simulink model "Iface"  (R2018b)
settings: Solver=FixedStepDiscrete  StartTime=0.0  StopTime=10.0  RelTol=1e-3
settings Model: Creator=matlab  LastModifiedBy=matlab
settings DataIOCC: SaveOutput=off  SignalLogging=off  SaveTime=off
settings OptimizationCC: DefaultParameterBehavior=Inlined  EnhancedBackFolding=on  PassReuseOutputArgsAs=Individual arguments  OptimizeBlockOrder=speed  DifferentSizesBufferReuse=on  OptimizationCustomize=off
settings DebuggingCC: ParameterTunabilityLossMsg=error
settings SFSimCC: MATLABDynamicMemAlloc=off
settings RTWCC: SystemTargetFile=ert.tlc  TemplateMakefile=ert_default_tmf  PostCodeGenCommand=packNGo(buildInfo);  GenerateReport=on  IncludeHyperlinkInReport=on  LaunchReport=on  GenerateTraceInfo=on  GenerateTraceReport=on  GenerateTraceReportSl=on  GenerateTraceReportSf=on  GenerateTraceReportEml=on
settings CodeAppCC: ForceParamTrailComments=on  IgnoreCustomStorageClasses=off  OperatorAnnotations=on  SimulinkDataObjDesc=on  SFDataObjDesc=on  InsertBlockDesc=on
settings ERTTargetCC: TargetLangStandard=C99 (ISO)  GenerateSampleERTMain=on  InlinedParameterPlacement=NonHierarchical  ERTCustomFileTemplate=example_file_process.tlc

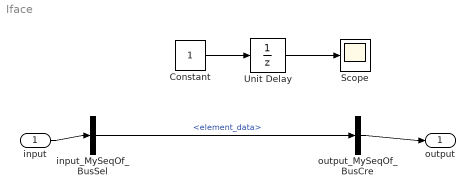
== system Iface ==
  input : Inport  OutDataTypeStr=Bus: MySeqOf  BusOutputAsStruct=on
  Constant : Constant
  Scope : Scope
  Unit Delay : UnitDelay  SampleTime=-1
  input_MySeqOf_BusSel : BusSelector  OutputSignals=element_data
  output_MySeqOf_BusCre : BusCreator  Inputs=1  OutDataTypeStr=Bus: MySeqOf  NonVirtualBus=on
  output : Outport  OutDataTypeStr=Bus: MySeqOf  BusOutputAsStruct=on
  wires:
  input/1 -> input_MySeqOf_BusSel/1
  output_MySeqOf_BusCre/1 -> output/1
  input_MySeqOf_BusSel/1 -> output_MySeqOf_BusCre/1  "<element_data>"
  Unit Delay/1 -> Scope/1
  Constant/1 -> Unit Delay/1
